simulink model "untitled"  (Simulink 7.7)
settings: Solver=ode3  StartTime=0.0  StopTime=200  RelTol=1e-3
libraries: dsparch4 x2, simulink x1
settings Model: Creator=Windows User  LastModifiedBy=Windows User

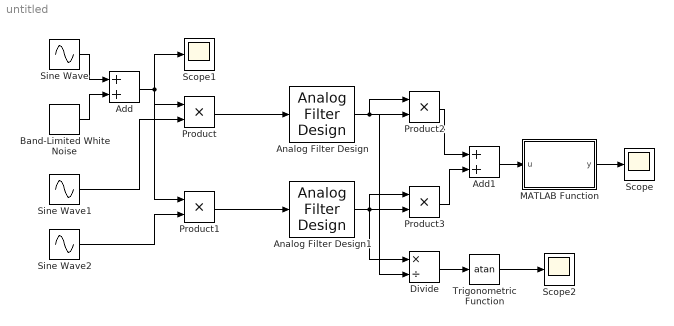
== system untitled ==
  Add : Sum
  Add1 : Sum
  Analog Filter Design : dsparch4/Analog Filter Design  method=Butterworth  filttype=Lowpass  N=8  Wlo=0.1  Whi=80  Rp=2  Rs=40
  Analog Filter Design1 : dsparch4/Analog Filter Design  method=Butterworth  filttype=Lowpass  N=8  Wlo=0.1  Whi=80  Rp=2  Rs=40
  Band-Limited White Noise : simulink/Sources/Band-Limited White Noise  SystemSampleTime=-1  Cov=[0.1]  Ts=0.1  seed=[23341]
  Divide : Product  Inputs=*/
  MATLAB Function : Stateflow chart  TreatAsAtomicUnit=on
  Product{,1..3} (4 alike) : Product  RndMeth=Zero
  Scope : Scope
  Scope1 : Scope
  Scope2 : Scope
      settings: SaveName=ScopeData2
  Sine Wave : Sin  Frequency=30*2*pi  Phase=pi/6  SampleTime=0
  Sine Wave1 : Sin  Frequency=30*pi*2  SampleTime=0
  Sine Wave2 : Sin  Phase=-pi/2  SampleTime=0
  Trigonometric Function : Trigonometry  Operator=atan
  wires:
  Sine Wave/1 -> Add/1
  Band-Limited White Noise/1 -> Add/2
  Add/1 -> Product/1, Scope1/1, Product1/1
  Product/1 -> Analog Filter Design/1
  Product1/1 -> Analog Filter Design1/1
  Analog Filter Design1/1 -> Product3/1, Product3/2, Divide/1
  Analog Filter Design/1 -> Product2/1, Product2/2, Divide/2
  Product3/1 -> Add1/2
  Product2/1 -> Add1/1
  Add1/1 -> MATLAB Function/1(u)
  Divide/1 -> Trigonometric Function/1
  MATLAB Function/1(y) -> Scope/1
  Trigonometric Function/1 -> Scope2/1
  Sine Wave1/1 -> Product/2
  Sine Wave2/1 -> Product1/2

== matlab function MATLAB Function ==
  data: u input double; y output double
function y = fcn(u)
%#codegen
y=2*sqrt(u)
